simulink model "EISGov_Governor"  (R2016b)
settings: configuration reference "CodeGenConfigSet" (kept outside this file)
values from neighbouring files (symbols this model uses):
  EISGov_bEngSPDropRestrainEN_C = Calibration.Parameter    [init_EISGov_Governor.m]    (also in init_EISGov_Governor_SIL.m = Simulink.Parameter)
  EISGov_DKd_CUR = Calibration.Parameter    [init_EISGov_Governor.m]    (also in init_EISGov_Governor_SIL.m = Simulink.Parameter)
  EISGov_DKd_CURX = Calibration.Parameter    [init_EISGov_Governor.m]    (also in init_EISGov_Governor_SIL.m = Simulink.Parameter)
  EISGov_dnDiffHi_C = Calibration.Parameter    [init_EISGov_Governor.m]    (also in init_EISGov_Governor_SIL.m = Simulink.Parameter)
  EISGov_dnDiffLo_C = Calibration.Parameter    [init_EISGov_Governor.m]    (also in init_EISGov_Governor_SIL.m = Simulink.Parameter)
  EISGov_facDT1_CUR = Calibration.Parameter    [init_EISGov_Governor.m]    (also in init_EISGov_Governor_SIL.m = Simulink.Parameter)
  EISGov_facDT1_CURX = Calibration.Parameter    [init_EISGov_Governor.m]    (also in init_EISGov_Governor_SIL.m = Simulink.Parameter)
  EISGov_facPT1DiffLoFlt_C = Calibration.Parameter    [init_EISGov_Governor.m]    (also in init_EISGov_Governor_SIL.m = Simulink.Parameter)
  EISGov_facPT1TrqFlt_CUR = Calibration.Parameter    [init_EISGov_Governor.m]    (also in init_EISGov_Governor_SIL.m = Simulink.Parameter)
  EISGov_facPT1TrqFlt_CURX = Calibration.Parameter    [init_EISGov_Governor.m]    (also in init_EISGov_Governor_SIL.m = Simulink.Parameter)
  EISGov_nDHypDenom_C = Calibration.Parameter    [init_EISGov_Governor.m]    (also in init_EISGov_Governor_SIL.m = Simulink.Parameter)
  EISGov_nDHypNum_C = Calibration.Parameter    [init_EISGov_Governor.m]    (also in init_EISGov_Governor_SIL.m = Simulink.Parameter)
  EISGov_nDiffHi_C = Calibration.Parameter    [init_EISGov_Governor.m]    (also in init_EISGov_Governor_SIL.m = Simulink.Parameter)
  EISGov_nDiffHiLim_C = Calibration.Parameter    [init_EISGov_Governor.m]    (also in init_EISGov_Governor_SIL.m = Simulink.Parameter)
  EISGov_nDiffLo_C = Calibration.Parameter    [init_EISGov_Governor.m]    (also in init_EISGov_Governor_SIL.m = Simulink.Parameter)
  EISGov_stDTSlect_C = Calibration.Parameter    [init_EISGov_Governor.m]    (also in init_EISGov_Governor_SIL.m = Simulink.Parameter)
  EISGov_stIInitDemChange_C = Calibration.Parameter    [init_EISGov_Governor.m]    (also in init_EISGov_Governor_SIL.m = Simulink.Parameter)
  EISGov_swtTrqFltNeg_C = Calibration.Parameter    [init_EISGov_Governor.m]    (also in init_EISGov_Governor_SIL.m = Simulink.Parameter)
  EISGov_tiDT1_CUR = Calibration.Parameter    [init_EISGov_Governor.m]    (also in init_EISGov_Governor_SIL.m = Simulink.Parameter)
  EISGov_tiDT1_CURX = Calibration.Parameter    [init_EISGov_Governor.m]    (also in init_EISGov_Governor_SIL.m = Simulink.Parameter)
  EISGov_tiTimeSPDropResActive_CUR = Calibration.Parameter    [init_EISGov_Governor.m]    (also in init_EISGov_Governor_SIL.m = Simulink.Parameter)
  EISGov_tiTimeSPDropResActive_CURX = Calibration.Parameter    [init_EISGov_Governor.m]    (also in init_EISGov_Governor_SIL.m = Simulink.Parameter)
  EISGov_trqIHiLimMax_C = Calibration.Parameter    [init_EISGov_Governor.m]    (also in init_EISGov_Governor_SIL.m = Simulink.Parameter)
  EISGov_trqIHiLimMin_C = Calibration.Parameter    [init_EISGov_Governor.m]    (also in init_EISGov_Governor_SIL.m = Simulink.Parameter)
  EISGov_trqILoLimMax_C = Calibration.Parameter    [init_EISGov_Governor.m]    (also in init_EISGov_Governor_SIL.m = Simulink.Parameter)
  EISGov_trqILoLimMin_C = Calibration.Parameter    [init_EISGov_Governor.m]    (also in init_EISGov_Governor_SIL.m = Simulink.Parameter)
  EISGov_trqPIHiLimMax_C = Calibration.Parameter    [init_EISGov_Governor.m]    (also in init_EISGov_Governor_SIL.m = Simulink.Parameter)
  EISGov_trqPIHiLimMin_C = Calibration.Parameter    [init_EISGov_Governor.m]    (also in init_EISGov_Governor_SIL.m = Simulink.Parameter)
  EISGov_trqPILoLimMax_C = Calibration.Parameter    [init_EISGov_Governor.m]    (also in init_EISGov_Governor_SIL.m = Simulink.Parameter)
  EISGov_trqPILoLimMin_C = Calibration.Parameter    [init_EISGov_Governor.m]    (also in init_EISGov_Governor_SIL.m = Simulink.Parameter)
  LIGov_numTempSel_C = Calibration.Parameter    [init_EISGov_Governor.m]    (also in init_EISGov_Governor_SIL.m = Simulink.Parameter)
undefined symbols (not defined in the file or in its folder): EISGov_Governor_DT, EpmSynState_conv, HLSDem_KpCorFac_MAPX, I_S16, nseLib, Switch_conv
libraries: simulink x28, CXLib x15
(part 1 of 2)
settings Model: Creator=Administrator  LastModifiedBy=xuxingpei
settings ConfigSetRef: SourceLocation=Base Workspace

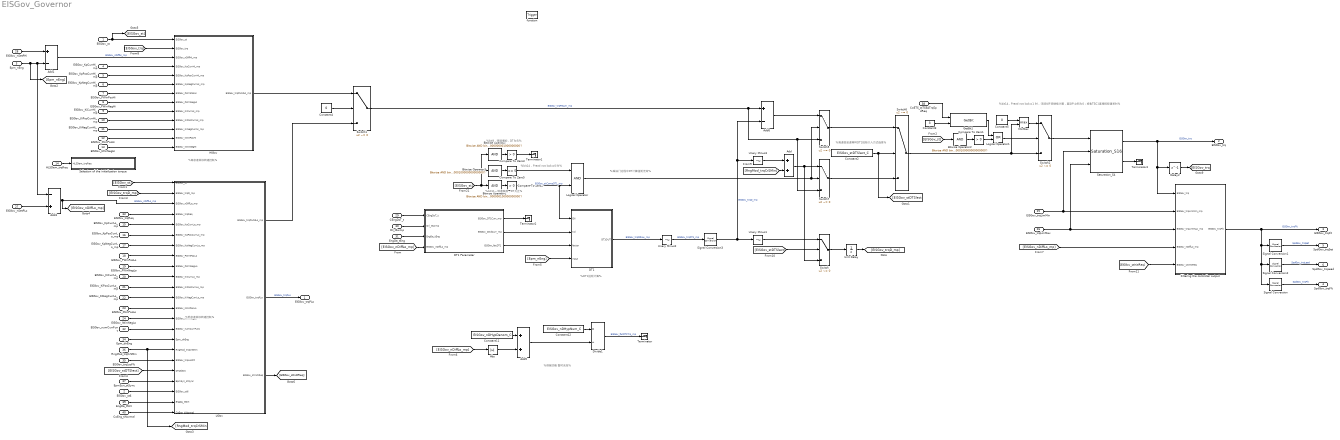
== system EISGov_Governor ==
  note: %保留功能 暂时无效%
  note: %高速回怠速两种DT1扭矩介入方式选择%
  note: %DT1扭矩计算%
  note: %踩油门过程中DT计算扭矩无效%
  note: %bit14，Prectl not lock=0 时%
  note: %bit9，转速增加，DT为负%
  note: %高怠速目标转速控制%
  note: %bit11，转速跌落，DT为正%
  note: %bit14，Prectl not lock=1 时，I项冻结P项继续计算，直到PI之和为0；或者TSC1直接扭矩请求时%
  note: %低怠速目标转速控制%
  EISGov_st : Inport  Description=Status information of EISGov and its clients  OutMin=0  OutMax=2147483648  OutDataTypeStr=State_uint32
  EISGov_st6 : Inport  Description=Status information of ExtDem client  Port=2  OutMin=0  OutMax=2147483648  OutDataTypeStr=State_uint32
  Epm_nEng : Inport  Tag=rpm  Description=Engine speed  Port=3  OutMin=0  OutMax=6000  OutDataTypeStr=EngSpeed_rpm
  EISGov_KpCurrHi_mp : Inport  Tag=Nm/rpm  Description=Current gain for the P element for the upper path  Port=4  OutMin=-10000  OutMax=10000  OutDataTypeStr=HLSDem_Kp
  EISGov_KpPosCurrHi_mp : Inport  Tag=Nm/rpm  Description=Current positive large signal gain for the P component upper PI-path  Port=5  OutMin=-10000  OutMax=10000  OutDataTypeStr=HLSDem_Kp
  EISGov_KpNegCurrHi_mp : Inport  Tag=Nm/rpm  Description=Current negative large signal gain for the P component upper PI-path  Port=6  OutMin=-10000  OutMax=10000  OutDataTypeStr=HLSDem_Kp
  EISGov_PWinPosHi : Inport  Tag=rpm  Description=P component Positive window for parameterset upper PI- path  Port=7  OutMin=-6000  OutMax=6000  OutDataTypeStr=EngSpeed_rpm
  EISGov_PWinNegHi : Inport  Tag=rpm  Description=P component negative window for parameterset upper PI- path  Port=8  OutMin=-6000  OutMax=6000  OutDataTypeStr=EngSpeed_rpm
  EISGov_KiCurrHi_mp : Inport  Tag=Nm/(rpm*s)  Description=Current gain for the I element for the upper path  Port=9  OutMin=-18000  OutMax=18000  OutDataTypeStr=HLSDem_Ki
  EISGov_KiPosCurrHi_mp : Inport  Tag=Nm/(rpm*s)  Description=Current positive large signal gain for the I component upper PI-path  Port=10  OutMin=-18000  OutMax=18000  OutDataTypeStr=HLSDem_Ki
  EISGov_KiNegCurrHi_mp : Inport  Tag=Nm/(rpm*s)  Description=Current negative large signal gain for the I component upper PI-path  Port=11  OutMin=-18000  OutMax=18000  OutDataTypeStr=HLSDem_Ki
  EISGov_IWinPosHi : Inport  Tag=rpm  Description=I component Positive window for parameterset upper PI- path  Port=12  OutMin=-6000  OutMax=6000  OutDataTypeStr=EngSpeed_rpm
  EISGov_IWinNegHi : Inport  Tag=rpm  Description=I component negative window for parameterset upper PI- path  Port=13  OutMin=-6000  OutMax=6000  OutDataTypeStr=EngSpeed_rpm
  HLSDem_trqReq : Inport  Tag=Nm  Description=Requested initialisation torque to engine speed governor (with reference to the output)  Port=14  OutMin=-3000  OutMax=3000  OutDataTypeStr=Trq_Nm
  EISGov_KpCurrLo_mp : Inport  Tag=Nm/rpm  Description=Current gain for the P element for the lower path  Port=15  OutMin=-10000  OutMax=10000  OutDataTypeStr=HLSDem_Kp
  EISGov_KpPosCurrLo_mp : Inport  Tag=Nm/rpm  Description=Current positive large signal gain for the P component lower PI-path  Port=16  OutMin=-10000  OutMax=10000  OutDataTypeStr=HLSDem_Kp
  EISGov_KpNegCurrLo_mp : Inport  Tag=Nm/rpm  Description=Current negative large signal gain for the P component lower PI-path  Port=17  OutMin=-10000  OutMax=10000  OutDataTypeStr=HLSDem_Kp
  EISGov_PWinPosLo : Inport  Tag=rpm  Description=P component Positive window for parameterset lower PI- path  Port=18  OutMin=-6000  OutMax=6000  OutDataTypeStr=EngSpeed_rpm
  EISGov_PWinNegLo : Inport  Tag=rpm  Description=P component negative window for parameterset lower PI- path  Port=19  OutMin=-6000  OutMax=6000  OutDataTypeStr=EngSpeed_rpm
  EISGov_KiCurrLo_mp : Inport  Tag=Nm/(rpm*s)  Description=Current gain for the I element for the lower path  Port=20  OutMin=-18000  OutMax=18000  OutDataTypeStr=HLSDem_Ki
  EISGov_KiPosCurrLo_mp : Inport  Tag=Nm/(rpm*s)  Description=Current positive large signal gain for the I component lower PI-path  Port=21  OutMin=-18000  OutMax=18000  OutDataTypeStr=HLSDem_Ki
  EISGov_KiNegCurrLo_mp : Inport  Tag=Nm/(rpm*s)  Description=Current negative large signal gain for the I component lower PI-path  Port=22  OutMin=-18000  OutMax=18000  OutDataTypeStr=HLSDem_Ki
  EISGov_IWinPosLo : Inport  Tag=rpm  Description=I component Positive window for parameterset lower PI- path  Port=23  OutMin=-6000  OutMax=6000  OutDataTypeStr=EngSpeed_rpm
  EISGov_IWinNegLo : Inport  Tag=rpm  Description=I component negative window for parameterset lower PI- path  Port=24  OutMin=-6000  OutMax=6000  OutDataTypeStr=EngSpeed_rpm
  EISGov_trqLimMin : Inport  Tag=Nm  Description=lower torque control limit for EISGov  Port=25  OutMin=-3276.8  OutMax=3276.7  OutDataTypeStr=Trq_Nm
  EISGov_trqLimMax : Inport  Tag=Nm  Description=Upper torque control limit for EISGov  Port=26  OutMin=-3276.8  OutMax=3276.7  OutDataTypeStr=Trq_Nm
  EISGov_nSetPLo : Inport  Tag=rpm  Description=Lower limit of the speed interval (set point speed) of the EISGov  Port=27  OutMin=0  OutMax=6000  OutDataTypeStr=EngSpeed_rpm
  EISGov_nSetPHi : Inport  Tag=rpm  Description=Upper limit of the speed interval (maximum speed) of EISGov  Port=28  OutMin=0  OutMax=6000  OutDataTypeStr=EngSpeed_rpm
  CEngDsT_t : Inport  Tag=deg  Description=engine coolant temperature after filter  Port=29  OutMin=-200  OutMax=200  OutDataTypeStr=Temp_deg
  Oil_tSwmp : Inport  Tag=deg  Description=Oil temperature in oil sump  Port=30  OutMin=-50  OutMax=200  OutDataTypeStr=Temp_deg
  EngDa_tEng : Inport  Tag=deg  Description=Engine temperature  Port=31  OutMin=-1000  OutMax=1000  OutDataTypeStr=Temp_deg
  EISGov_numCurrFunc : Inport  Description=Identification name / number of the currently active EISGov client, which determines the current controller parameters  Port=32  OutDataTypeStr=Enum: EISGov_num_conv
  EISGov_trqReq : Inport  Tag=Nm  Description=Selected requirement (from all the requirements of the active EISGov clients) to the EISGov for an initialisation torque  Port=33  OutMin=-3276.8  OutMax=3276.7  OutDataTypeStr=Trq_Nm
  Epm_dnEng : Inport  Tag=rpm/s  Description=Engine speed gradient calculated over current crankshaft-segment (S0-S0 or S1-S1)  Port=34  OutMin=-12000  OutMax=12000  OutDataTypeStr=EngSpeed_rpm_s
  EISGov_trqLosFlt : Inport  Tag=Nm  Description=estimated torque loss  Port=35  OutMin=-3276.8  OutMax=3276.7  OutDataTypeStr=Trq_Nm
  RngMod_trqCrSMin : Inport  Tag=Nm  Description=minimal crankshaft torque  Port=36  OutMin=-3276.8  OutMax=3276.7  OutDataTypeStr=Trq_Nm
  EpmSyn_stSync : Inport  Description=state of synchronization  Port=37  OutDataTypeStr=Enum: EpmSynState_conv
  CoETS_stTSEATrqSpdReq : Inport  Description=Status of information about torque and speed intervention  Port=38  OutMin=0  OutMax=65535  OutDataTypeStr=State_uint16
  EngDa_tStrt : Inport  Tag=deg  Description=Engine starting temperature  Port=39  OutMin=-1000  OutMax=1000  OutDataTypeStr=Temp_deg
  CoEng_tiNormal : Inport  Tag=ms  Description="Time since state\"CONENG_RUNNING\"was reached"  Port=40  OutMin=0  OutMax=42949672950  OutDataTypeStr=EngTime_ms
  function : TriggerPort  TriggerType=function-call  VariantControl=Variant
  Abs : Abs
  Add : Sum  SaturateOnIntegerOverflow=on
  Add1 : Sum  Inputs=+-  SaturateOnIntegerOverflow=on  InputSameDT=on
  Add3 : Sum  Inputs=-+  SaturateOnIntegerOverflow=on  InputSameDT=on
  Add5 : Sum  SaturateOnIntegerOverflow=on  InputSameDT=on
  Add6 : Sum  Inputs=+-  SaturateOnIntegerOverflow=on  InputSameDT=on
  Bitwise Operator : simulink/Logic and Bit Operations/Bitwise Operator  logicop=AND  UseBitMask=on  BitMask=bin2dec('00000000000000000000001000000000')  BitMaskRealWorld=Stored Integer
  Bitwise Operator1 : simulink/Logic and Bit Operations/Bitwise Operator  logicop=AND  UseBitMask=on  BitMask=bin2dec('00000000000000000000100000000000')  BitMaskRealWorld=Stored Integer
  Bitwise Operator2 : simulink/Logic and Bit Operations/Bitwise Operator  logicop=AND  UseBitMask=on  BitMask=bin2dec('00000000000000000100000000000000')  BitMaskRealWorld=Stored Integer
  Bitwise Operator3 : simulink/Logic and Bit Operations/Bitwise Operator  logicop=AND  UseBitMask=on  BitMask=bin2dec('00000000000000000100000000000000')  BitMaskRealWorld=Stored Integer
  Compare To Zero1 : simulink/Logic and Bit Operations/Compare To Zero  relop=>  OutDataTypeStr=boolean
  Compare To Zero2 : simulink/Logic and Bit Operations/Compare To Zero  relop=>  OutDataTypeStr=boolean
  Compare To Zero3 : simulink/Logic and Bit Operations/Compare To Zero  relop=>  OutDataTypeStr=boolean
  Compare To Zero5 : simulink/Logic and Bit Operations/Compare To Zero  relop===  OutDataTypeStr=boolean
  Constant11 : Constant  Value=EISGov_nDHypDenom_C
  Constant12 : Constant  Value=EISGov_nDHypNum_C
  Constant2 : Constant  Value=EISGov_stDTSlect_C
  Constant3 : Constant  Value=3  OutDataTypeStr=Inherit: Inherit via back propagation
  Constant4 : Constant  Value=0  OutDataTypeStr=boolean
  Constant5 : Constant  Value=0  OutDataTypeStr=Inherit: Inherit via back propagation
  DT1 : Subsystem
  DT1 Parameter : Subsystem
  Delay2 : Delay  DelayLength=1  InitialCondition=0
  Divide1 : Product  Inputs=*/  OutDataTypeStr=Inherit: Inherit via back propagation  RndMeth=Round  SaturateOnIntegerOverflow=on
  Filtering the controller output : Subsystem
  GetBit1 : CXLib/GetBit  dataTypeString=uint16  dataLength=0
      settings: AttributesFormatString=Get bit from %<dataTypeString>
  HIGov : Subsystem
  LIGov : Subsystem
  Logical Operator : Logic  AllPortsSameDT=off  OutDataTypeStr=boolean
  Logical Operator1 : Logic  Operator=OR  AllPortsSameDT=off  OutDataTypeStr=boolean
  MinMax : MinMax  Function=max  Inputs=2  OutDataTypeStr=Inherit: Inherit via back propagation
  Saturation_S4 : CXLib/Saturation_S16
  "Selection of the initialization torque " : Subsystem
  Signal Conversion{,1..3} (4 alike) : SignalConversion  OverrideOpt=off
  Switch{,5..7} (4 alike) : Switch  Criteria=u2 ~= 0  OutDataTypeStr=Inherit: Inherit via back propagation
  Switch1 : Switch  Criteria=u2 ~= 0  InputSameDT=on
  Switch2 : Switch  Criteria=u2 ~= 0  InputSameDT=on
  Terminator{,1..2,4} (4 alike) : Terminator
  Unary Minus1 : UnaryMinus  SaturateOnIntegerOverflow=on
  Unary Minus2 : UnaryMinus  SaturateOnIntegerOverflow=on
  Unary Minus3 : UnaryMinus  SaturateOnIntegerOverflow=on
  Unit Delay : UnitDelay  SampleTime=-1
      settings: AttributesFormatString=InitialValue=%<InitialCondition>
  EISGov_trqPLo : Outport  Tag=Nm  Description=P-component of the lower path  OutMin=-3276.8  OutMax=3276.7  OutDataTypeStr=Trq_Nm
  EISGov_trq : Outport  Tag=Nm  Description=Resulted output torque of EISGov controller  Port=2  OutMin=-3276.8  OutMax=3276.7  OutDataTypeStr=Trq_Nm
  EISGov_trqFlt : Outport  Tag=Nm  Description=Filtered output torque of the EISGov  Port=3  OutMin=-3276.8  OutMax=3276.7  OutDataTypeStr=Trq_Nm
  SpdGov_trqFlt : Outport  Tag=Nm  Description=filtered setpoint torque of SpdGov  Port=4  OutMin=-3267  OutMax=3267  OutDataTypeStr=Trq_Nm
  SpdGov_trqSet : Outport  Tag=Nm  Description=Set point torque of SpdGov on the fuel path  Port=5  OutMin=-3000  OutMax=3000  OutDataTypeStr=Trq_Nm
  SpdGov_trqLead : Outport  Tag=Nm  Description=lead torque of SpdGov on the air path  Port=6  OutMin=-3267  OutMax=3267  OutDataTypeStr=Trq_Nm
  wires:
  Epm_nEng/1 -> [Epm_nEng], Add3/1, Add1/2
  EISGov_trqLimMin/1 -> Saturation_S4/2, Filtering the controller output/2(EISGov_trqLimMin_mp)
  EISGov_trqLimMax/1 -> Saturation_S4/3, Filtering the controller output/3(EISGov_trqLimMax_mp)
  Saturation_S4/2 -> Terminator4/1
  Filtering the controller output/1(EISGov_trqFlt) -> Signal Conversion2/1, Signal Conversion/1, Signal Conversion1/1, EISGov_trqFlt/1  "EISGov_trqFlt"
  Bitwise Operator/1 -> Compare To Zero3/1
  [EISGov_st] -> Bitwise Operator/1, Bitwise Operator3/1, Bitwise Operator1/1
  Bitwise Operator1/1 -> Compare To Zero2/1
  Abs/1 -> Add5/2
  Constant11/1 -> Add5/1
  Constant12/1 -> Divide1/1
  Add5/1 -> Divide1/2
  Divide1/1 -> Terminator/1  "EISGov_facDT1Trq_mp"
  EISGov_nSetPHi/1 -> Add1/1
  Add3/1 -> LIGov/3(EISGov_nDiffLo_mp), [EISGov_nDiffLo_mp]  "EISGov_nDiffLo_mp"
  EISGov_nSetPLo/1 -> Add3/2
  Add1/1 -> HIGov/3(EISGov_nDiffHi_mp)  "EISGov_nDiffHi_mp"
  EISGov_st/1 -> [EISGov_st], HIGov/1(EISGov_st)
  [EISGov_st] -> LIGov/1(EISGov_st)
  HIGov/1(EISGov_trqPILtdHi_mp) -> Switch1/1
  LIGov/1(EISGov_trqPILtdLo_mp) -> Switch1/3
  Constant4/1 -> Switch1/2
  [EISGov_nDiffLo_mp] -> Abs/1
  [EISGov_nDiffLo_mp] -> Filtering the controller output/4(EISGov_nDiffLo_mp)
  [EISGov_trq] -> HIGov/2(EISGov_trq)
  [EISGov_trqD_mp] -> LIGov/2(EISGov_trqD_mp)
  Saturation_S4/1 -> Delay2/1, Filtering the controller output/1(EISGov_trq), EISGov_trq/1  "EISGov_trq"
  Delay2/1 -> [EISGov_trq]
  EISGov_trqReq/1 -> LIGov/4(EISGov_trqReq)
  LIGov/2(EISGov_trqPLo) -> EISGov_trqPLo/1  "EISGov_trqPLo"
  Bitwise Operator2/1 -> Compare To Zero1/1
  [EISGov_st] -> Bitwise Operator2/1
  Compare To Zero2/1 -> DT1/1(EN), Logical Operator/2  "EISGov_stCompDT1_mp"
  Signal Conversion/1 -> SpdGov_trqFlt/1  "SpdGov_trqFlt"
  Signal Conversion2/1 -> SpdGov_trqLead/1  "SpdGov_trqLead"
  Signal Conversion1/1 -> SpdGov_trqSet/1  "SpdGov_trqSet"
  CEngDsT_t/1 -> DT1 Parameter/1(CEngDsT_t)
  Oil_tSwmp/1 -> DT1 Parameter/2(Oil_tSwmp)
  EngDa_tEng/1 -> DT1 Parameter/3(EngDa_tEng)
  EISGov_KpCurrHi_mp/1 -> HIGov/4(EISGov_KpCurrHi_mp)
  EISGov_KpPosCurrHi_mp/1 -> HIGov/5(EISGov_KpPosCurrHi_mp)
  EISGov_KpNegCurrHi_mp/1 -> HIGov/6(EISGov_KpNegCurrHi_mp)
  EISGov_PWinPosHi/1 -> HIGov/7(EISGov_PWinPosHi)
  EISGov_PWinNegHi/1 -> HIGov/8(EISGov_PWinNegHi)
  EISGov_KiCurrHi_mp/1 -> HIGov/9(EISGov_KiCurrHi_mp)
  EISGov_KiPosCurrHi_mp/1 -> HIGov/10(EISGov_KiPosCurrHi_mp)
  EISGov_KiNegCurrHi_mp/1 -> HIGov/11(EISGov_KiNegCurrHi_mp)
  EISGov_IWinPosHi/1 -> HIGov/12(EISGov_IWinPosHi)
  EISGov_IWinNegHi/1 -> HIGov/13(EISGov_IWinNegHi)
  EISGov_KpCurrLo_mp/1 -> LIGov/5(EISGov_KpCurrLo_mp)
  EISGov_KpPosCurrLo_mp/1 -> LIGov/6(EISGov_KpPosCurrLo_mp)
  EISGov_KpNegCurrLo_mp/1 -> LIGov/7(EISGov_KpNegCurrLo_mp)
  EISGov_PWinPosLo/1 -> LIGov/8(EISGov_PWinPosLo)
  EISGov_PWinNegLo/1 -> LIGov/9(EISGov_PWinNegLo)
  EISGov_KiCurrLo_mp/1 -> LIGov/10(EISGov_KiCurrLo_mp)
  EISGov_KiPosCurrLo_mp/1 -> LIGov/11(EISGov_KiPosCurrLo_mp)
  EISGov_KiNegCurrLo_mp/1 -> LIGov/12(EISGov_KiNegCurrLo_mp)
  EISGov_IWinPosLo/1 -> LIGov/13(EISGov_IWinPosLo)
  EISGov_IWinNegLo/1 -> LIGov/14(EISGov_IWinNegLo)
  Unit Delay/1 -> [EISGov_trqD_mp]
  HLSDem_trqReq/1 -> "Selection of the initialization torque "/1(HLSDem_trqReq)
  EISGov_numCurrFunc/1 -> LIGov/15(EISGov_numCurrFunc)
  Constant5/1 -> MinMax/1
  MinMax/1 -> Switch2/1
  Epm_dnEng/1 -> LIGov/16(Epm_dnEng)
  RngMod_trqCrSMin/1 -> LIGov/17(RngMod_trqCrSMin), [RngMod_trqCrSMin]
  EISGov_trqLosFlt/1 -> LIGov/18(EISGov_trqLosFlt)
  DT1 Parameter/2(EISGov_DKdCurr_mp) -> DT1/2(Kd)
  DT1/1(DT1OUT) -> Unary Minus2/1  "EISGov_trqDRaw_mp"
  Unary Minus2/1 -> Signal Conversion3/1  "EISGov_trqDT1_mp"
  Signal Conversion3/1 -> Unary Minus1/1, Add6/2, Unary Minus3/1  "EISGov_trqD_mp"
  Switch7/1 -> Switch6/3
  [EISGov_stDTSlect] -> LIGov/19(DT1Slect)
  Switch1/1 -> Switch5/3, Switch7/3, Add6/1  "EISGov_trqPISum_mp"
  Switch6/1 -> MinMax/2, Switch2/3
  Switch2/1 -> Saturation_S4/1
  Logical Operator/1 -> Switch5/2, Switch7/2
  Constant2/1 -> Switch6/2, [EISGov_stDTSlect]
  Switch5/1 -> Switch6/1
  Add6/1 -> Switch5/1
  Compare To Zero3/1 -> Terminator1/1
  DT1 Parameter/1(EISGov_DT1Curr_mp) -> Terminator2/1
  Bitwise Operator3/1 -> Compare To Zero5/1
  Compare To Zero5/1 -> Logical Operator/1
  [Epm_nEng] -> DT1/4(Input)
  [EISGov_nDiffLo_mp] -> DT1 Parameter/4(EISGov_nDiffLo_mp)
  DT1 Parameter/3(EISGov_facDT1) -> DT1/3(factor)
  Unary Minus1/1 -> Switch/1
  [EISGov_stDTSlect] -> Switch/2
  Add/1 -> Switch/3, Switch7/1
  [RngMod_trqCrSMin] -> Add/2
  Unary Minus3/1 -> Add/1
  Switch/1 -> Unit Delay/1
  EpmSyn_stSync/1 -> LIGov/20(EpmSyn_stSync)
  EISGov_st6/1 -> LIGov/21(EISGov_st6)
  GetBit1/1 -> Logical Operator1/1
  Constant3/1 -> GetBit1/2
  CoETS_stTSEATrqSpdReq/1 -> GetBit1/1
  Compare To Zero1/1 -> Logical Operator1/2
  Logical Operator1/1 -> Switch2/2
  EngDa_tStrt/1 -> LIGov/22(EngDa_tStrt)
  CoEng_tiNormal/1 -> LIGov/23(CoEng_tiNormal)
  LIGov/3(EISGov_stInitIReq) -> [EISGov_stInitIReq]
  [EISGov_stInitIReq] -> Filtering the controller output/5(EISGov_stInitIReq)

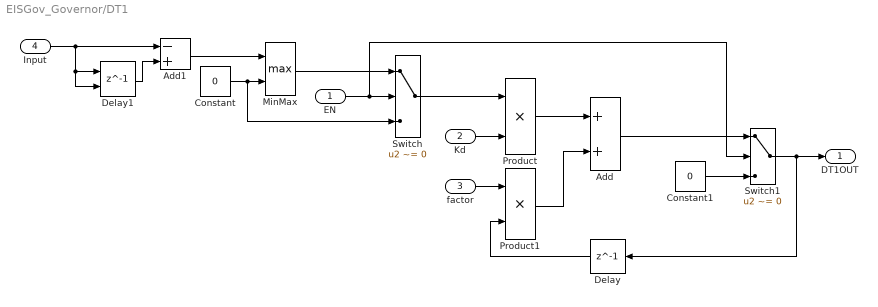
== system EISGov_Governor/DT1 ==
  EN : Inport
  Kd : Inport  Port=2
  factor : Inport  Port=3
  Input : Inport  Port=4
  Add : Sum  OutDataTypeStr=Inherit: Inherit via back propagation  SaturateOnIntegerOverflow=on
  Add1 : Sum  Inputs=-+  OutDataTypeStr=Inherit: Inherit via back propagation  SaturateOnIntegerOverflow=on  InputSameDT=on
  Constant : Constant  Value=0  OutDataTypeStr=Inherit: Inherit via back propagation
  Constant1 : Constant  Value=0  OutDataTypeStr=Inherit: Inherit via back propagation
  Delay : Delay  DelayLength=1  InitialCondition=0
  Delay1 : Delay  DelayLength=1  InitialConditionSource=Input port  InitialCondition=0
      settings: InputPortMap=u0,p4
  MinMax : MinMax  Function=max  Inputs=2
  Product : Product  OutDataTypeStr=fixdt(1,32,0.0001,0)  SaturateOnIntegerOverflow=on
  Product1 : Product  OutDataTypeStr=fixdt(1,32,0.0001,0)  SaturateOnIntegerOverflow=on
  Switch : Switch  Criteria=u2 ~= 0  OutDataTypeStr=Inherit: Inherit via back propagation
  Switch1 : Switch  Criteria=u2 ~= 0  InputSameDT=on
  DT1OUT : Outport
  wires:
  Kd/1 -> Product/2
  Product/1 -> Add/1
  Add/1 -> Switch1/1
  Constant/1 -> Switch/3, MinMax/2
  Delay/1 -> Product1/2
  Product1/1 -> Add/2
  factor/1 -> Product1/1
  Input/1 -> Add1/1, Delay1/1, Delay1/2
  Delay1/1 -> Add1/2
  Add1/1 -> MinMax/1
  EN/1 -> Switch1/2, Switch/2
  MinMax/1 -> Switch/1
  Switch/1 -> Product/1
  Constant1/1 -> Switch1/3
  Switch1/1 -> Delay/1, DT1OUT/1

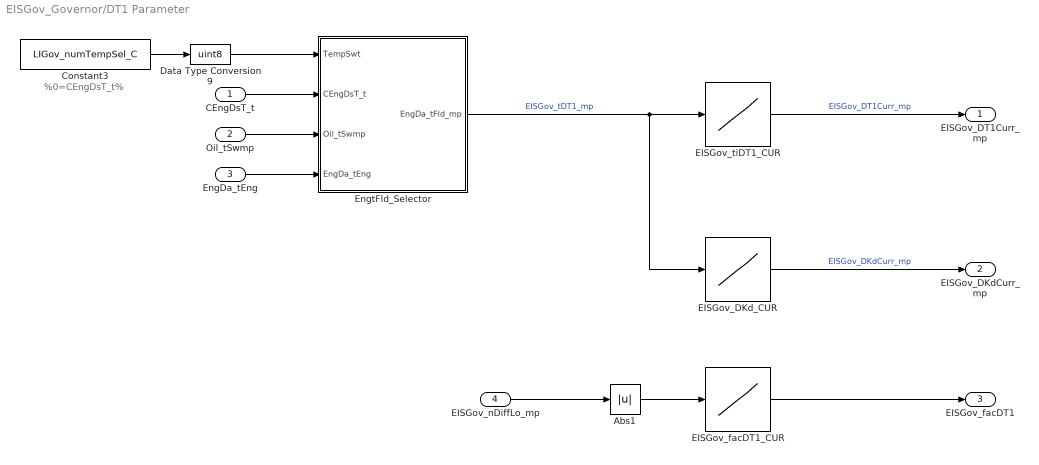
== system EISGov_Governor/DT1 Parameter ==
  note: %0=CEngDsT_t%
  CEngDsT_t : Inport  Tag=deg  Description=engine coolant temperature after filter  OutMin=-200  OutMax=200  OutDataTypeStr=Temp_deg
  Oil_tSwmp : Inport  Tag=deg  Description=Oil temperature in oil sump  Port=2  OutMin=-50  OutMax=200  OutDataTypeStr=Temp_deg
  EngDa_tEng : Inport  Tag=deg  Description=Engine temperature  Port=3  OutMin=-1000  OutMax=1000  OutDataTypeStr=Temp_deg
  EISGov_nDiffLo_mp : Inport  Port=4
  Abs1 : Abs
  Constant3 : Constant  Value=LIGov_numTempSel_C
  Data Type Conversion9 : DataTypeConversion  OutDataTypeStr=uint8
  EISGov_DKd_CUR : Lookup_n-D  NumberOfTableDimensions=1  BreakpointsForDimension1=EISGov_DKd_CURX  Table=EISGov_DKd_CUR  ExtrapMethod=Clip  InternalRulePriority=Speed  OutDataTypeStr=Inherit: Inherit via back propagation  RndMeth=Simplest  SaturateOnIntegerOverflow=on
  EISGov_facDT1_CUR : Lookup_n-D  NumberOfTableDimensions=1  BreakpointsForDimension1=EISGov_facDT1_CURX  Table=EISGov_facDT1_CUR  ExtrapMethod=Clip  InternalRulePriority=Speed  OutDataTypeStr=Inherit: Inherit via back propagation  RndMeth=Simplest  SaturateOnIntegerOverflow=on
  EISGov_tiDT1_CUR : Lookup_n-D  NumberOfTableDimensions=1  BreakpointsForDimension1=EISGov_tiDT1_CURX  Table=EISGov_tiDT1_CUR  ExtrapMethod=Clip  InternalRulePriority=Speed  OutDataTypeStr=Inherit: Inherit via back propagation  RndMeth=Simplest  SaturateOnIntegerOverflow=on
  EngtFld_Selector : Subsystem
  EISGov_DT1Curr_mp : Outport
  EISGov_DKdCurr_mp : Outport  Port=2
  EISGov_facDT1 : Outport  Port=3
  wires:
  EISGov_tiDT1_CUR/1 -> EISGov_DT1Curr_mp/1  "EISGov_DT1Curr_mp"
  Constant3/1 -> Data Type Conversion9/1
  EngtFld_Selector/1(EngDa_tFld_mp) -> EISGov_DKd_CUR/1, EISGov_tiDT1_CUR/1  "EISGov_tDT1_mp"
  EISGov_DKd_CUR/1 -> EISGov_DKdCurr_mp/1  "EISGov_DKdCurr_mp"
  Data Type Conversion9/1 -> EngtFld_Selector/1(TempSwt)
  CEngDsT_t/1 -> EngtFld_Selector/2(CEngDsT_t)
  Oil_tSwmp/1 -> EngtFld_Selector/3(Oil_tSwmp)
  EngDa_tEng/1 -> EngtFld_Selector/4(EngDa_tEng)
  Abs1/1 -> EISGov_facDT1_CUR/1
  EISGov_facDT1_CUR/1 -> EISGov_facDT1/1
  EISGov_nDiffLo_mp/1 -> Abs1/1

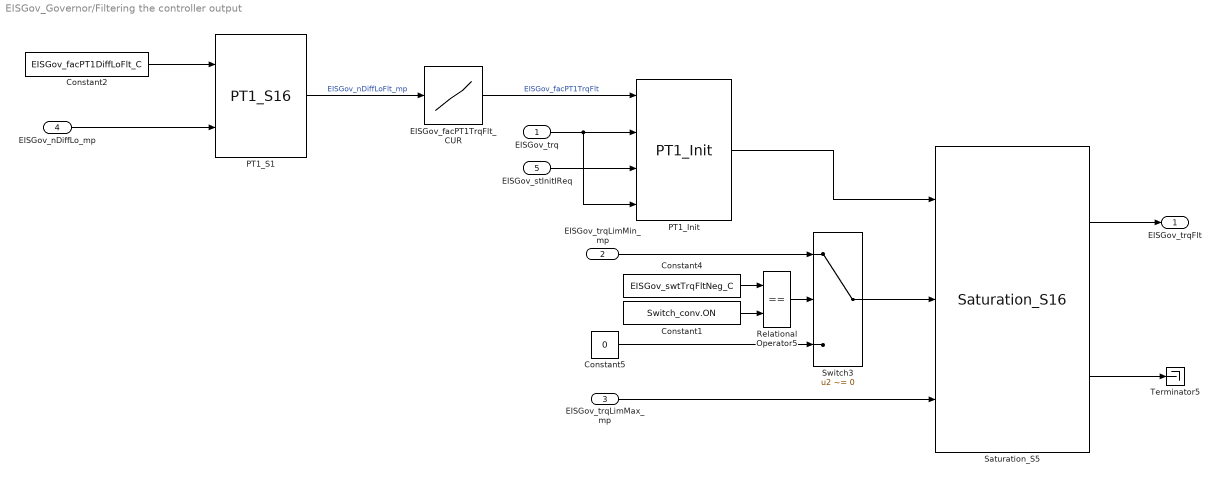
== system EISGov_Governor/Filtering the controller output ==
  EISGov_trq : Inport
  EISGov_trqLimMin_mp : Inport  Port=2
  EISGov_trqLimMax_mp : Inport  Port=3
  EISGov_nDiffLo_mp : Inport  Port=4
  EISGov_stInitIReq : Inport  Port=5
  Constant1 : Constant  Value=Switch_conv.ON  OutDataTypeStr=Inherit: Inherit via back propagation
  Constant2 : Constant  Value=EISGov_facPT1DiffLoFlt_C
  Constant4 : Constant  Value=EISGov_swtTrqFltNeg_C
  Constant5 : Constant  Value=0  OutDataTypeStr=Inherit: Inherit via back propagation
  EISGov_facPT1TrqFlt_CUR : Lookup_n-D  NumberOfTableDimensions=1  BreakpointsForDimension1=EISGov_facPT1TrqFlt_CURX  Table=EISGov_facPT1TrqFlt_CUR  ExtrapMethod=Clip  InternalRulePriority=Speed  OutDataTypeStr=Inherit: Inherit via back propagation  RndMeth=Simplest  SaturateOnIntegerOverflow=on
  PT1_Init : CXLib/PT1_Init
  PT1_S1 : CXLib/PT1_S16
  Relational Operator5 : RelationalOperator  Operator===  OutDataTypeStr=boolean  RndMeth=Simplest  InputSameDT=on
  Saturation_S5 : CXLib/Saturation_S16
  Switch3 : Switch  Criteria=u2 ~= 0  InputSameDT=on
  Terminator5 : Terminator
  EISGov_trqFlt : Outport
  wires:
  EISGov_trq/1 -> PT1_Init/4, PT1_Init/2
  EISGov_trqLimMax_mp/1 -> Saturation_S5/3
  EISGov_trqLimMin_mp/1 -> Switch3/1
  PT1_Init/1 -> Saturation_S5/1
  Saturation_S5/1 -> EISGov_trqFlt/1
  Saturation_S5/2 -> Terminator5/1
  Switch3/1 -> Saturation_S5/2
  Constant5/1 -> Switch3/3
  Relational Operator5/1 -> Switch3/2
  Constant4/1 -> Relational Operator5/1
  Constant1/1 -> Relational Operator5/2
  EISGov_facPT1TrqFlt_CUR/1 -> PT1_Init/1  "EISGov_facPT1TrqFlt"
  PT1_S1/1 -> EISGov_facPT1TrqFlt_CUR/1  "EISGov_nDiffLoFlt_mp"
  Constant2/1 -> PT1_S1/1
  EISGov_nDiffLo_mp/1 -> PT1_S1/2
  EISGov_stInitIReq/1 -> PT1_Init/3

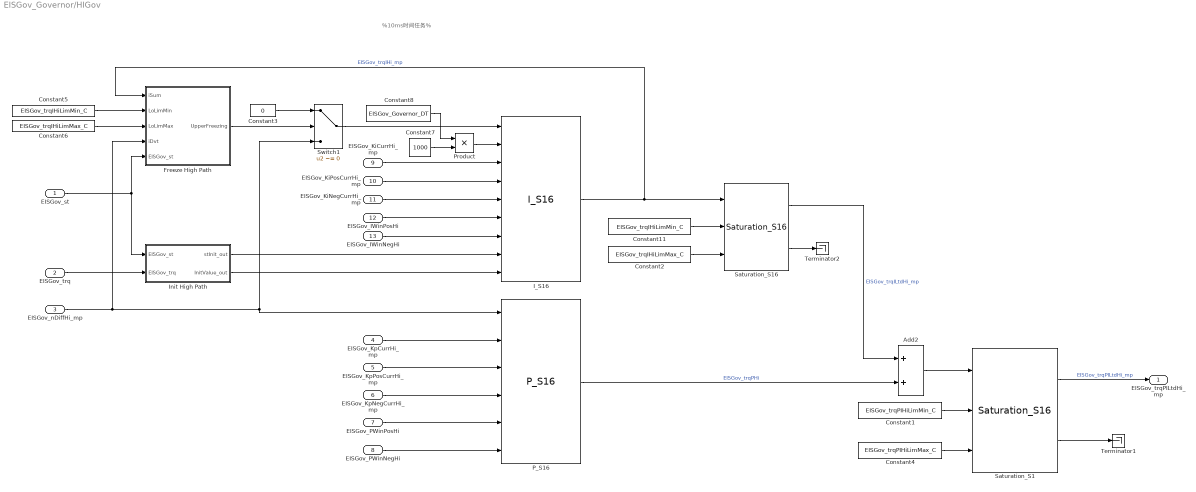
== system EISGov_Governor/HIGov ==
  note: %10ms时间任务%
  EISGov_st : Inport
  EISGov_trq : Inport  Port=2
  EISGov_nDiffHi_mp : Inport  Port=3
  EISGov_KpCurrHi_mp : Inport  Tag=Nm/rpm  Description=Current gain for the P element for the upper path  Port=4  OutMin=-10000  OutMax=10000  OutDataTypeStr=HLSDem_Kp
  EISGov_KpPosCurrHi_mp : Inport  Tag=Nm/rpm  Description=Current positive large signal gain for the P component upper PI-path  Port=5  OutMin=-10000  OutMax=10000  OutDataTypeStr=HLSDem_Kp
  EISGov_KpNegCurrHi_mp : Inport  Tag=Nm/rpm  Description=Current negative large signal gain for the P component upper PI-path  Port=6  OutMin=-10000  OutMax=10000  OutDataTypeStr=HLSDem_Kp
  EISGov_PWinPosHi : Inport  Tag=rpm  Description=P component Positive window for parameterset upper PI- path  Port=7  OutMin=-6000  OutMax=6000  OutDataTypeStr=EngSpeed_rpm
  EISGov_PWinNegHi : Inport  Tag=rpm  Description=P component negative window for parameterset upper PI- path  Port=8  OutMin=-6000  OutMax=6000  OutDataTypeStr=EngSpeed_rpm
  EISGov_KiCurrHi_mp : Inport  Tag=Nm/(rpm*s)  Description=Current gain for the I element for the upper path  Port=9  OutMin=-18000  OutMax=18000  OutDataTypeStr=HLSDem_Ki
  EISGov_KiPosCurrHi_mp : Inport  Tag=Nm/(rpm*s)  Description=Current positive large signal gain for the I component upper PI-path  Port=10  OutMin=-18000  OutMax=18000  OutDataTypeStr=HLSDem_Ki
  EISGov_KiNegCurrHi_mp : Inport  Tag=Nm/(rpm*s)  Description=Current negative large signal gain for the I component upper PI-path  Port=11  OutMin=-18000  OutMax=18000  OutDataTypeStr=HLSDem_Ki
  EISGov_IWinPosHi : Inport  Tag=rpm  Description=I component Positive window for parameterset upper PI- path  Port=12  OutMin=-6000  OutMax=6000  OutDataTypeStr=EngSpeed_rpm
  EISGov_IWinNegHi : Inport  Tag=rpm  Description=I component negative window for parameterset upper PI- path  Port=13  OutMin=-6000  OutMax=6000  OutDataTypeStr=EngSpeed_rpm
  Add2 : Sum  SaturateOnIntegerOverflow=on  InputSameDT=on
  Constant1 : Constant  Value=EISGov_trqPIHiLimMin_C
  Constant11 : Constant  Value=EISGov_trqIHiLimMin_C
  Constant2 : Constant  Value=EISGov_trqIHiLimMax_C
  Constant3 : Constant  Value=0  OutDataTypeStr=Inherit: Inherit via back propagation
  Constant4 : Constant  Value=EISGov_trqPIHiLimMax_C
  Constant5 : Constant  Value=EISGov_trqIHiLimMin_C
  Constant6 : Constant  Value=EISGov_trqIHiLimMax_C
  Constant7 : Constant  Value=1000  OutDataTypeStr=Inherit: Inherit via back propagation
  Constant8 : Constant  Value=EISGov_Governor_DT  OutDataTypeStr=Inherit: Inherit via back propagation
  Freeze High Path : Subsystem
  I_S16 : CXLib/I_S16
  Init High Path : Subsystem
  P_S16 : CXLib/P_S16
  Product : Product  OutDataTypeStr=uint32
  Saturation_S1 : CXLib/Saturation_S16
  Saturation_S16 : CXLib/Saturation_S16
  Switch1 : Switch  Criteria=u2 ~= 0  InputSameDT=on
  Terminator1 : Terminator
  Terminator2 : Terminator
  EISGov_trqPILtdHi_mp : Outport
  wires:
  EISGov_trq/1 -> Init High Path/2(EISGov_trq)
  EISGov_nDiffHi_mp/1 -> P_S16/1, Switch1/3, Freeze High Path/4(iDvt)
  P_S16/1 -> Add2/2  "EISGov_trqPHi"
  I_S16/1 -> Freeze High Path/1(iSum), Saturation_S16/1  "EISGov_trqIHi_mp"
  Saturation_S16/1 -> Add2/1  "EISGov_trqILtdHi_mp"
  Add2/1 -> Saturation_S1/1
  Saturation_S1/2 -> Terminator1/1
  Saturation_S1/1 -> EISGov_trqPILtdHi_mp/1  "EISGov_trqPILtdHi_mp"
  Constant3/1 -> Switch1/1
  Init High Path/1(stInit_out) -> I_S16/8
  EISGov_PWinNegHi/1 -> P_S16/6
  EISGov_PWinPosHi/1 -> P_S16/5
  EISGov_KpNegCurrHi_mp/1 -> P_S16/4
  EISGov_KpPosCurrHi_mp/1 -> P_S16/3
  EISGov_KpCurrHi_mp/1 -> P_S16/2
  Freeze High Path/1(UpperFreezing) -> Switch1/2
  EISGov_st/1 -> Freeze High Path/5(EISGov_st), Init High Path/1(EISGov_st)
  Constant11/1 -> Saturation_S16/2
  Constant2/1 -> Saturation_S16/3
  Saturation_S16/2 -> Terminator2/1
  Constant6/1 -> Freeze High Path/3(LoLimMax)
  Constant5/1 -> Freeze High Path/2(LoLimMin)
  Constant1/1 -> Saturation_S1/2
  Constant4/1 -> Saturation_S1/3
  Switch1/1 -> I_S16/1
  EISGov_KiCurrHi_mp/1 -> I_S16/3
  EISGov_KiPosCurrHi_mp/1 -> I_S16/4
  EISGov_KiNegCurrHi_mp/1 -> I_S16/5
  EISGov_IWinPosHi/1 -> I_S16/6
  EISGov_IWinNegHi/1 -> I_S16/7
  Init High Path/2(InitValue_out) -> I_S16/9
  Constant7/1 -> Product/2
  Product/1 -> I_S16/2
  Constant8/1 -> Product/1

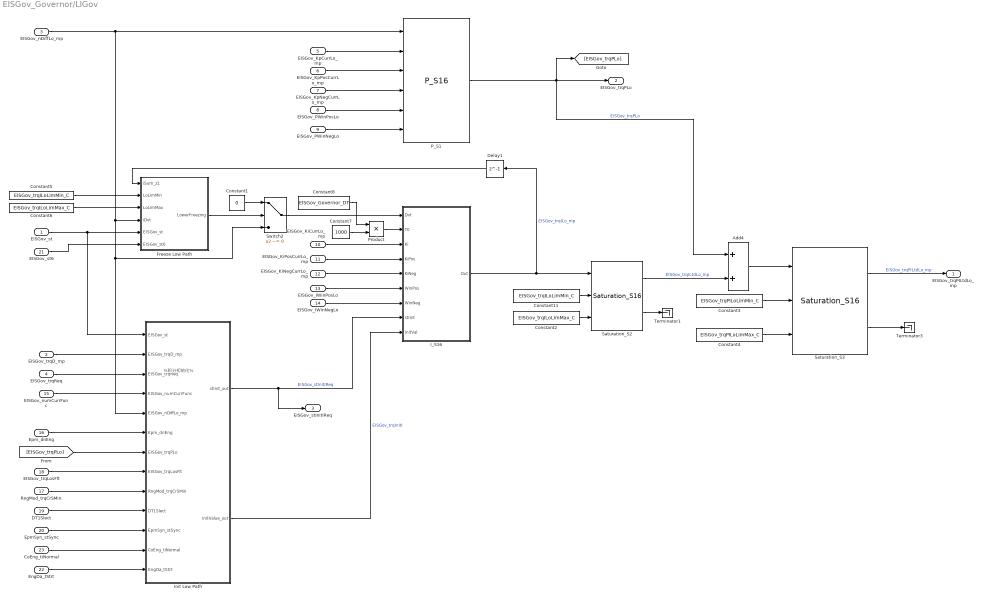
== system EISGov_Governor/LIGov ==
  note: %积分初始化%
  EISGov_st : Inport
  EISGov_trqD_mp : Inport  Port=2
  EISGov_nDiffLo_mp : Inport  Port=3
  EISGov_trqReq : Inport  Port=4
  EISGov_KpCurrLo_mp : Inport  Tag=Nm/rpm  Description=Current gain for the P element for the lower path  Port=5  OutMin=-10000  OutMax=10000  OutDataTypeStr=HLSDem_Kp
  EISGov_KpPosCurrLo_mp : Inport  Tag=Nm/rpm  Description=Current positive large signal gain for the P component lower PI-path  Port=6  OutMin=-10000  OutMax=10000  OutDataTypeStr=HLSDem_Kp
  EISGov_KpNegCurrLo_mp : Inport  Tag=Nm/rpm  Description=Current negative large signal gain for the P component lower PI-path  Port=7  OutMin=-10000  OutMax=10000  OutDataTypeStr=HLSDem_Kp
  EISGov_PWinPosLo : Inport  Tag=rpm  Description=P component Positive window for parameterset lower PI- path  Port=8  OutMin=-6000  OutMax=6000  OutDataTypeStr=EngSpeed_rpm
  EISGov_PWinNegLo : Inport  Tag=rpm  Description=P component negative window for parameterset lower PI- path  Port=9  OutMin=-6000  OutMax=6000  OutDataTypeStr=EngSpeed_rpm
  EISGov_KiCurrLo_mp : Inport  Tag=Nm/(rpm*s)  Description=Current gain for the I element for the lower path  Port=10  OutMin=-18000  OutMax=18000  OutDataTypeStr=HLSDem_Ki
  EISGov_KiPosCurrLo_mp : Inport  Tag=Nm/(rpm*s)  Description=Current positive large signal gain for the I component lower PI-path  Port=11  OutMin=-18000  OutMax=18000  OutDataTypeStr=HLSDem_Ki
  EISGov_KiNegCurrLo_mp : Inport  Tag=Nm/(rpm*s)  Description=Current negative large signal gain for the I component lower PI-path  Port=12  OutMin=-18000  OutMax=18000  OutDataTypeStr=HLSDem_Ki
  EISGov_IWinPosLo : Inport  Tag=rpm  Description=I component Positive window for parameterset lower PI- path  Port=13  OutMin=-6000  OutMax=6000  OutDataTypeStr=EngSpeed_rpm
  EISGov_IWinNegLo : Inport  Tag=rpm  Description=I component negative window for parameterset lower PI- path  Port=14  OutMin=-6000  OutMax=6000  OutDataTypeStr=EngSpeed_rpm
  EISGov_numCurrFunc : Inport  Description=Identification name / number of the currently active EISGov client, which determines the current controller parameters  Port=15  OutDataTypeStr=Enum: EISGov_num_conv
  Epm_dnEng : Inport  Tag=rpm/s  Description=Engine speed gradient calculated over current crankshaft-segment (S0-S0 or S1-S1)  Port=16  OutMin=-12000  OutMax=12000  OutDataTypeStr=EngSpeed_rpm_s
  RngMod_trqCrSMin : Inport  Port=17
  EISGov_trqLosFlt : Inport  Port=18
  DT1Slect : Inport  Port=19
  EpmSyn_stSync : Inport  Port=20
  EISGov_st6 : Inport  Port=21
  EngDa_tStrt : Inport  Description=state of starting system  Port=22
  CoEng_tiNormal : Inport  Tag=ms  Description="Time since state\"CONENG_RUNNING\"was reached"  Port=23
  Add4 : Sum  SaturateOnIntegerOverflow=on  InputSameDT=on
  Constant1 : Constant  Value=0  OutDataTypeStr=Inherit: Inherit via back propagation
  Constant11 : Constant  Value=EISGov_trqILoLimMin_C
  Constant2 : Constant  Value=EISGov_trqILoLimMax_C
  Constant3 : Constant  Value=EISGov_trqPILoLimMin_C
  Constant4 : Constant  Value=EISGov_trqPILoLimMax_C
  Constant5 : Constant  Value=EISGov_trqILoLimMin_C
  Constant6 : Constant  Value=EISGov_trqILoLimMax_C
  Constant7 : Constant  Value=1000  OutDataTypeStr=Inherit: Inherit via back propagation
  Constant8 : Constant  Value=EISGov_Governor_DT  OutDataTypeStr=Inherit: Inherit via back propagation
  Delay1 : Delay  DelayLength=1  InitialCondition=0
  Freeze Low Path : Subsystem
  I_S16 : Subsystem  AncestorBlock=nseLib/I_S16  TreatAsAtomicUnit=on  RTWFcnName=lib_I_S16  RTWFileName=service_library  mask(I_S16){}
      mask help:
      | Ki模块：一般用于计算结果的累加,该模块多用于SCR模块；
      | WinNeg<=Dvt<=WinPos,  Yout=Ylast+Ki*Dvt
      | Dvt>WinPos         ,  Yout=Ylast+KiPos*Dvt
      | Dvt<WinNeg         ,  Yout=Ylast+KiNeg*Dvt
      |
      | In1（由使用情况定）: Dvt,控制对象偏差（x/s）；
      | In2（uint32）: T0，采样时间（us）；
      | In3（Pid_Ki）: Ki，窗口内的Ki系数（默认为1）；
      | In4（Pid_Ki）: KiPos，上限窗口的Ki系数（默认为1）；
      | In5（Pid_Ki）: KiNeg，下限窗口的Ki系数（默认为1）；
      | In6（由使用情况定）: WinPos，上窗口阀值；
      | In6（由使用情况定）: WinNeg，下窗口阀值；
      | In7（boolean）: stInit，初始化使能端口；
      | In8（由使用情况定）: InitVal，初始化值(x)；
      |
      | Out1（由使用情况定）: Out
      mask Display: image('IControl.jpg')
  Init Low Path : Subsystem
  P_S1 : CXLib/P_S16
  Product : Product  OutDataTypeStr=uint32
  Saturation_S2 : CXLib/Saturation_S16
  Saturation_S3 : CXLib/Saturation_S16
  Switch2 : Switch  Criteria=u2 ~= 0  InputSameDT=on
  Terminator1 : Terminator
  Terminator3 : Terminator
  EISGov_trqPILtdLo_mp : Outport
  EISGov_trqPLo : Outport  Port=2
  EISGov_stInitIReq : Outport  Port=3
  wires:
  EISGov_trqD_mp/1 -> Init Low Path/2(EISGov_trqD_mp)
  EISGov_nDiffLo_mp/1 -> Init Low Path/5(EISGov_nDiffLo_mp), Switch2/3, Freeze Low Path/4(iDvt), P_S1/1
  Switch2/1 -> I_S16/1(Dvt)
  Constant1/1 -> Switch2/1
  Init Low Path/1(stInit_out) -> I_S16/8(stInit), EISGov_stInitIReq/1  "EISGov_stInitIReq"
  Init Low Path/2(InitValue_out) -> I_S16/9(InitVal)  "EISGov_trqInitI"
  I_S16/1(Out) -> Delay1/1, Saturation_S2/1  "EISGov_trqILo_mp"
  Saturation_S2/1 -> Add4/2  "EISGov_trqILtdLo_mp"
  P_S1/1 -> [EISGov_trqPLo], Add4/1, EISGov_trqPLo/1  "EISGov_trqPLo"
  Add4/1 -> Saturation_S3/1
  Saturation_S3/2 -> Terminator3/1
  Saturation_S3/1 -> EISGov_trqPILtdLo_mp/1  "EISGov_trqPILtdLo_mp"
  EISGov_KiNegCurrLo_mp/1 -> I_S16/5(KiNeg)
  EISGov_KiPosCurrLo_mp/1 -> I_S16/4(KiPos)
  EISGov_KiCurrLo_mp/1 -> I_S16/3(Ki)
  EISGov_PWinNegLo/1 -> P_S1/6
  EISGov_PWinPosLo/1 -> P_S1/5
  EISGov_KpNegCurrLo_mp/1 -> P_S1/4
  EISGov_KpPosCurrLo_mp/1 -> P_S1/3
  EISGov_KpCurrLo_mp/1 -> P_S1/2
  EISGov_IWinPosLo/1 -> I_S16/6(WinPos)
  EISGov_IWinNegLo/1 -> I_S16/7(WinNeg)
  Freeze Low Path/1(LowerFreezing) -> Switch2/2
  EISGov_st/1 -> Init Low Path/1(EISGov_st), Freeze Low Path/5(EISGov_st)
  Constant11/1 -> Saturation_S2/2
  Constant2/1 -> Saturation_S2/3
  Saturation_S2/2 -> Terminator1/1
  Constant6/1 -> Freeze Low Path/3(LoLimMax)
  Constant5/1 -> Freeze Low Path/2(LoLimMin)
  Constant3/1 -> Saturation_S3/2
  Constant4/1 -> Saturation_S3/3
  EISGov_trqReq/1 -> Init Low Path/3(EISGov_trqReq)
  Product/1 -> I_S16/2(T0)
  Constant7/1 -> Product/2
  Constant8/1 -> Product/1
  Delay1/1 -> Freeze Low Path/1(iSum_z1)
  EISGov_numCurrFunc/1 -> Init Low Path/4(EISGov_numCurrFunc)
  [EISGov_trqPLo] -> Init Low Path/7(EISGov_trqPLo)
  Epm_dnEng/1 -> Init Low Path/6(Epm_dnEng)
  RngMod_trqCrSMin/1 -> Init Low Path/9(RngMod_trqCrSMin)
  EISGov_trqLosFlt/1 -> Init Low Path/8(EISGov_trqLosFlt)
  DT1Slect/1 -> Init Low Path/10(DT1Slect)
  EpmSyn_stSync/1 -> Init Low Path/11(EpmSyn_stSync)
  EISGov_st6/1 -> Freeze Low Path/6(EISGov_st6)
  EngDa_tStrt/1 -> Init Low Path/13(EngDa_tStrt)
  CoEng_tiNormal/1 -> Init Low Path/12(CoEng_tiNormal)

== system EISGov_Governor/Selection of the initialization torque  ==
  HLSDem_trqReq : Inport
  Terminator : Terminator
  wires:
  HLSDem_trqReq/1 -> Terminator/1

== system EISGov_Governor/DT1 Parameter/EngtFld_Selector ==
  TempSwt : Inport
  CEngDsT_t : Inport  Tag=deg  Description=engine coolant temperature after filter  Port=2
  Oil_tSwmp : Inport  Tag=deg  Description=Oil temperature in oil sump  Port=3
  EngDa_tEng : Inport  Tag=deg  Description=Engine temperature  Port=4
  Data Type Conversion : DataTypeConversion  OutDataTypeStr=uint8
  Multiport Switch : MultiPortSwitch  DataPortOrder=Zero-based contiguous
  EngDa_tFld_mp : Outport  Tag=deg  Description=Engine temperature field
  wires:
  CEngDsT_t/1 -> Multiport Switch/2
  Multiport Switch/1 -> EngDa_tFld_mp/1
  EngDa_tEng/1 -> Multiport Switch/4
  Oil_tSwmp/1 -> Multiport Switch/3
  Data Type Conversion/1 -> Multiport Switch/1
  TempSwt/1 -> Data Type Conversion/1

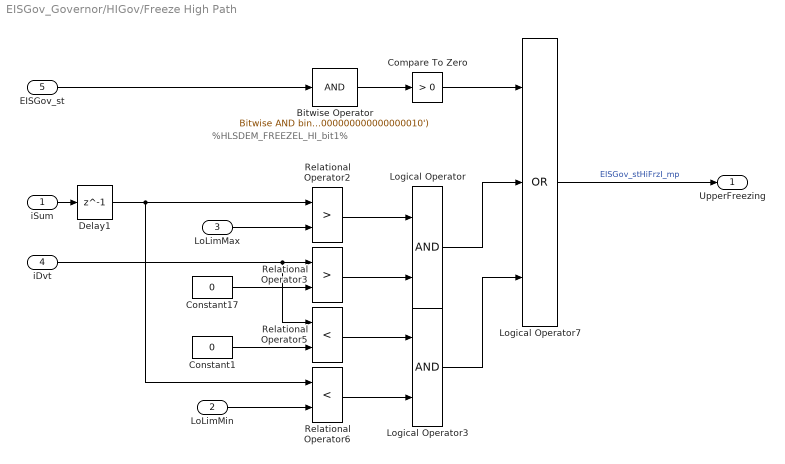
== system EISGov_Governor/HIGov/Freeze High Path ==
  note: %HLSDEM_FREEZEL_HI_bit1%
  iSum : Inport
  LoLimMin : Inport  Port=2
  LoLimMax : Inport  Port=3
  iDvt : Inport  Port=4
  EISGov_st : Inport  Port=5
  Bitwise Operator : simulink/Logic and Bit Operations/Bitwise Operator  logicop=AND  UseBitMask=on  BitMask=bin2dec('00000000000000000000000000000010')  BitMaskRealWorld=Stored Integer
  Compare To Zero : simulink/Logic and Bit Operations/Compare To Zero  relop=>  OutDataTypeStr=boolean
  Constant1 : Constant  Value=0  OutDataTypeStr=Inherit: Inherit via back propagation  SampleTime=-1
  Constant17 : Constant  Value=0  OutDataTypeStr=Inherit: Inherit via back propagation  SampleTime=-1
  Delay1 : Delay  DelayLength=1  InitialCondition=0
  Logical Operator : Logic  AllPortsSameDT=off  OutDataTypeStr=boolean
  Logical Operator3 : Logic  AllPortsSameDT=off  OutDataTypeStr=boolean
  Logical Operator7 : Logic  Operator=OR  Inputs=3  OutDataTypeStr=boolean
  Relational Operator2 : RelationalOperator  Operator=>  OutDataTypeStr=boolean  RndMeth=Nearest  InputSameDT=on
  Relational Operator3 : RelationalOperator  Operator=>  OutDataTypeStr=boolean  RndMeth=Nearest  InputSameDT=on
  Relational Operator5 : RelationalOperator  Operator=<  OutDataTypeStr=boolean  RndMeth=Nearest  InputSameDT=on
  Relational Operator6 : RelationalOperator  Operator=<  OutDataTypeStr=boolean  RndMeth=Nearest  InputSameDT=on
  UpperFreezing : Outport
  wires:
  EISGov_st/1 -> Bitwise Operator/1
  Bitwise Operator/1 -> Compare To Zero/1
  Logical Operator7/1 -> UpperFreezing/1  "EISGov_stHiFrzI_mp"
  Relational Operator6/1 -> Logical Operator3/2
  Relational Operator5/1 -> Logical Operator3/1
  Relational Operator3/1 -> Logical Operator/2
  Relational Operator2/1 -> Logical Operator/1
  LoLimMin/1 -> Relational Operator6/2
  Constant17/1 -> Relational Operator3/2
  iDvt/1 -> Relational Operator5/1, Relational Operator3/1
  iSum/1 -> Delay1/1
  LoLimMax/1 -> Relational Operator2/2
  Constant1/1 -> Relational Operator5/2
  Logical Operator/1 -> Logical Operator7/2
  Logical Operator3/1 -> Logical Operator7/3
  Compare To Zero/1 -> Logical Operator7/1
  Delay1/1 -> Relational Operator6/1, Relational Operator2/1

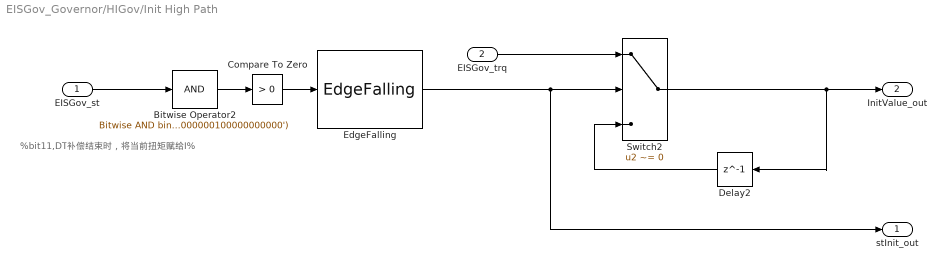
== system EISGov_Governor/HIGov/Init High Path ==
  note: %bit11,DT补偿结束时，将当前扭矩赋给I%
  EISGov_st : Inport
  EISGov_trq : Inport  Port=2
  Bitwise Operator2 : simulink/Logic and Bit Operations/Bitwise Operator  logicop=AND  UseBitMask=on  BitMask=bin2dec('00000000000000000000100000000000')  BitMaskRealWorld=Stored Integer
  Compare To Zero : simulink/Logic and Bit Operations/Compare To Zero  relop=>  OutDataTypeStr=boolean
  Delay2 : Delay  DelayLength=1  InitialCondition=0
  EdgeFalling : CXLib/EdgeFalling
  Switch2 : Switch  Criteria=u2 ~= 0  InputSameDT=on
  stInit_out : Outport
  InitValue_out : Outport  Port=2
  wires:
  Switch2/1 -> InitValue_out/1, Delay2/1
  EISGov_trq/1 -> Switch2/1
  EISGov_st/1 -> Bitwise Operator2/1
  Bitwise Operator2/1 -> Compare To Zero/1
  EdgeFalling/1 -> stInit_out/1, Switch2/2
  Delay2/1 -> Switch2/3
  Compare To Zero/1 -> EdgeFalling/1

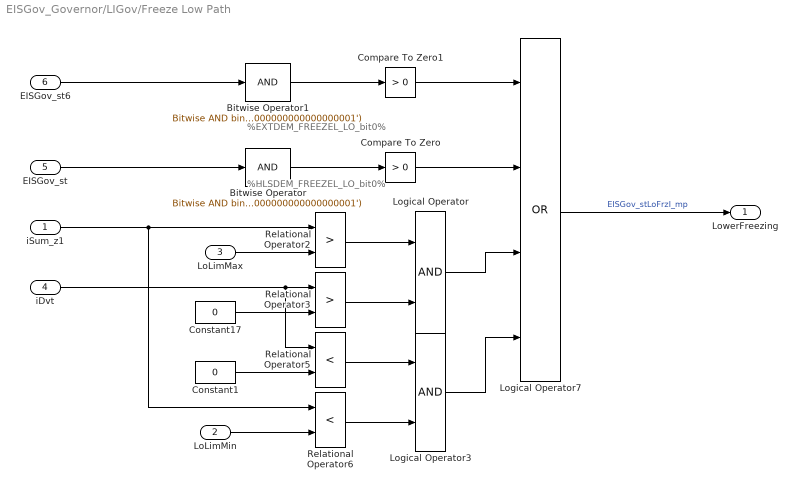
== system EISGov_Governor/LIGov/Freeze Low Path ==
  note: %HLSDEM_FREEZEL_LO_bit0%
  note: %EXTDEM_FREEZEL_LO_bit0%
  iSum_z1 : Inport
  LoLimMin : Inport  Port=2
  LoLimMax : Inport  Port=3
  iDvt : Inport  Port=4
  EISGov_st : Inport  Port=5
  EISGov_st6 : Inport  Port=6
  Bitwise Operator : simulink/Logic and Bit Operations/Bitwise Operator  logicop=AND  UseBitMask=on  BitMask=bin2dec('00000000000000000000000000000001')  BitMaskRealWorld=Stored Integer
  Bitwise Operator1 : simulink/Logic and Bit Operations/Bitwise Operator  logicop=AND  UseBitMask=on  BitMask=bin2dec('00000000000000000000000000000001')  BitMaskRealWorld=Stored Integer
  Compare To Zero : simulink/Logic and Bit Operations/Compare To Zero  relop=>  OutDataTypeStr=boolean
  Compare To Zero1 : simulink/Logic and Bit Operations/Compare To Zero  relop=>  OutDataTypeStr=boolean
  Constant1 : Constant  Value=0  OutDataTypeStr=Inherit: Inherit via back propagation  SampleTime=-1
  Constant17 : Constant  Value=0  OutDataTypeStr=Inherit: Inherit via back propagation  SampleTime=-1
  Logical Operator : Logic  AllPortsSameDT=off  OutDataTypeStr=boolean
  Logical Operator3 : Logic  AllPortsSameDT=off  OutDataTypeStr=boolean
  Logical Operator7 : Logic  Operator=OR  Inputs=4  OutDataTypeStr=boolean
  Relational Operator2 : RelationalOperator  Operator=>  OutDataTypeStr=boolean  RndMeth=Nearest  InputSameDT=on
  Relational Operator3 : RelationalOperator  Operator=>  OutDataTypeStr=boolean  RndMeth=Nearest  InputSameDT=on
  Relational Operator5 : RelationalOperator  Operator=<  OutDataTypeStr=boolean  RndMeth=Nearest  InputSameDT=on
  Relational Operator6 : RelationalOperator  Operator=<  OutDataTypeStr=boolean  RndMeth=Nearest  InputSameDT=on
  LowerFreezing : Outport
  wires:
  EISGov_st/1 -> Bitwise Operator/1
  Bitwise Operator/1 -> Compare To Zero/1
  Logical Operator7/1 -> LowerFreezing/1  "EISGov_stLoFrzI_mp"
  Relational Operator6/1 -> Logical Operator3/2
  Relational Operator5/1 -> Logical Operator3/1
  Relational Operator3/1 -> Logical Operator/2
  Relational Operator2/1 -> Logical Operator/1
  LoLimMin/1 -> Relational Operator6/2
  Constant17/1 -> Relational Operator3/2
  iDvt/1 -> Relational Operator5/1, Relational Operator3/1
  LoLimMax/1 -> Relational Operator2/2
  Constant1/1 -> Relational Operator5/2
  iSum_z1/1 -> Relational Operator6/1, Relational Operator2/1
  EISGov_st6/1 -> Bitwise Operator1/1
  Logical Operator3/1 -> Logical Operator7/4
  Logical Operator/1 -> Logical Operator7/3
  Compare To Zero/1 -> Logical Operator7/2
  Bitwise Operator1/1 -> Compare To Zero1/1
  Compare To Zero1/1 -> Logical Operator7/1

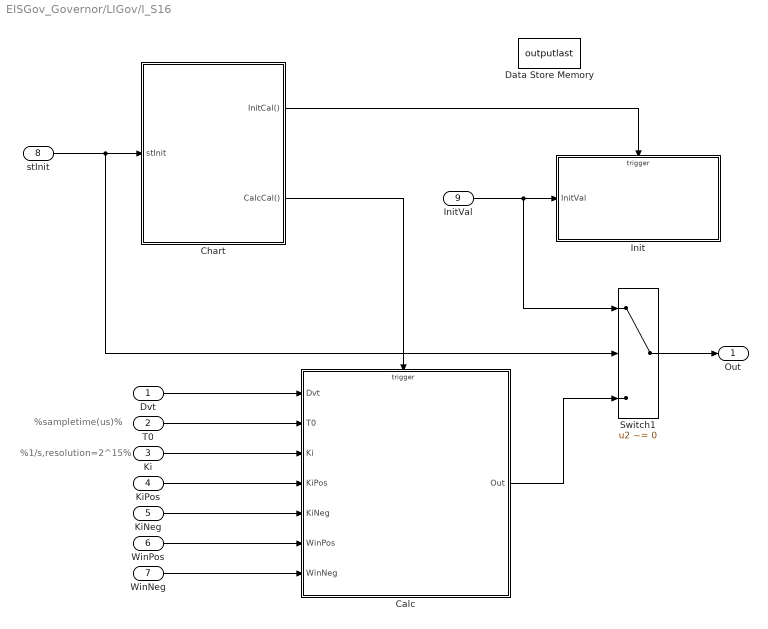
== system EISGov_Governor/LIGov/I_S16 ==
  note: %sampletime(us)%
  note: %1/s,resolution=2^15%
  Dvt : Inport
  T0 : Inport  Port=2  OutDataTypeStr=uint32
  Ki : Inport  Port=3
  KiPos : Inport  Port=4
  KiNeg : Inport  Port=5
  WinPos : Inport  Port=6
  WinNeg : Inport  Port=7
  stInit : Inport  Port=8  OutDataTypeStr=boolean
  InitVal : Inport  Port=9
  Calc : Subsystem
  Chart : Stateflow chart  TreatAsAtomicUnit=on
  Data Store Memory : DataStoreMemory  DataStoreName=outputlast  ReadBeforeWriteMsg=warning  WriteAfterWriteMsg=warning  WriteAfterReadMsg=warning  ShowAdditionalParam=off  OutDataTypeStr=fixdt(1,32,0.001,0)
  Init : Subsystem  TreatAsAtomicUnit=on
  Switch1 : Switch  Criteria=u2 ~= 0  SaturateOnIntegerOverflow=on  InputSameDT=on
  Out : Outport
  wires:
  Switch1/1 -> Out/1
  Chart/2(CalcCal()) -> Calc/Trigger
  Calc/1(Out) -> Switch1/3
  Ki/1 -> Calc/3(Ki)
  WinNeg/1 -> Calc/7(WinNeg)
  KiNeg/1 -> Calc/5(KiNeg)
  T0/1 -> Calc/2(T0)
  WinPos/1 -> Calc/6(WinPos)
  KiPos/1 -> Calc/4(KiPos)
  Dvt/1 -> Calc/1(Dvt)
  InitVal/1 -> Init/1(InitVal), Switch1/1
  Chart/1(InitCal()) -> Init/Trigger
  stInit/1 -> Chart/1(stInit), Switch1/2
